simulink model "ServidorConNovint"  (Simulink 8.3)
settings: Solver=FixedStepDiscrete  StartTime=0.0  StopTime=inf  FixedStep=0.001  RelTol=1e-3
libraries: aerolibanimutils x1
settings Model: Creator=Usuario  LastModifiedBy=DdS
settings OptimizationCC: ExpressionDepthLimit=2147483647  SimCompilerOptimization=On
settings DebuggingCC: FcnCallInpInsideContextMsg=EnableAllAsWarning

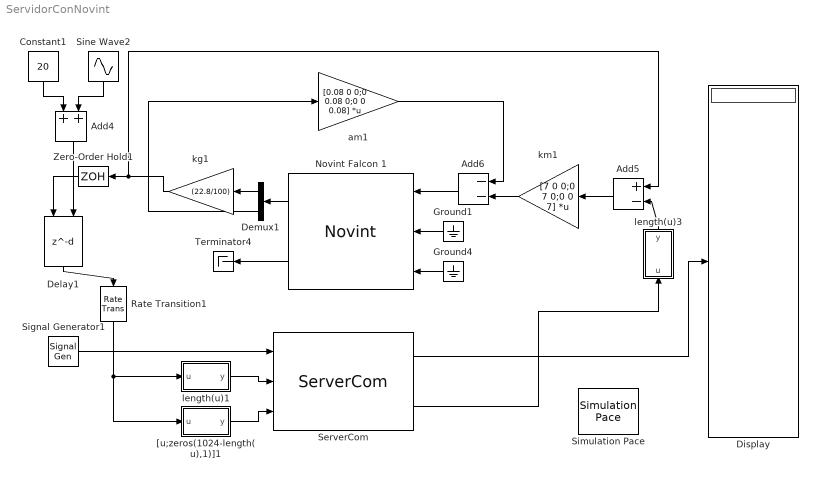
== system ServidorConNovint ==
  Add4 : Sum  SampleTime=0.05
  Add5 : Sum  Inputs=+-
  Add6 : Sum  Inputs=--
  Constant1 : Constant  Value=20  SampleTime=0.05
  Delay1 : Delay  DelayLengthSource=Input port  SampleTime=0.05
      settings: InputPortMap=u0,p1
  Demux1 : Demux  Outputs=[3 3]
  Display : Display
  Ground1 : Ground
  Ground4 : Ground
  Novint Falcon 1 : S-Function  FunctionName=Novint  Parameters=1  EnableBusSupport=off
      mask Display:
      | color('red')
      | port_label('input',1,'acciones')
      | port_label('input',2,'parametros')
      | port_label('input',3,'parametrosSend')
      | color('blue')
      | port_label('output',1,'estado')
      | port_label('output',2,'botones')
  Rate Transition1 : RateTransition  OutPortSampleTime=0
  ServerCom : S-Function  FunctionName=ServerCom  EnableBusSupport=off
      mask Display:
      | patch([0 4. 4 0],[0.02 0.02 0.98 0.98],0.9*[123 193 255]/255)
      | patch([0 4 4 0],[0.1 0.1 0.9 0.9],[123 193 255]/255)
      | patch([1.5 2.5 2.5 2.3 2.3 1.7 1.7 1.5],[0 0 1 1 1.2 1.2 1 1],[130 130 130]/255)
      | patch([1.3 2.7 2.7 1.3],[1.2 1.2 2.9 2.9],0.85*[130 130 130]/255)
      | patch([1.4 2.6 2.6 1.4],[1.3 1.3 2.8 2.8],[123 193 255]/255)
      | patch([1.5 2.5 2.5 1.5],[1.4 1.4 2.7 2.7],0.85*[130 130 130]/255)
      | patch([1.9 2.1 2.1 1.9],[1.8 1.8 2.1 2.1],[123 193 255]/255)
      | color('red')
      | port_label('input',1,'clock')
      | port_label('input',2,'sizeSend')
      | port_label('input',3,'dataSend')
      | port_label('output',1,'stateChannel')
      | port_label('output',2,'dataRecv')
  Signal Generator1 : SignalGenerator  WaveForm=square  Frequency=20
  Simulation Pace : aerolibanimutils/Simulation Pace  SimulationPace=1  SleepMode=MATLAB Thread  OutputPaceError=off  SampleTime=-1
      settings: AttributesFormatString=%<SimulationPace> sec/sec
  Sine Wave2 : Sin  Amplitude=0  Frequency=0.1*2*pi  SampleTime=0.05
  Terminator4 : Terminator
  Zero-Order Hold1 : ZeroOrderHold  SampleTime=0.05
  "[u;zeros(1024-length(u),1)]1" : MATLAB Function  TreatAsAtomicUnit=on
  am1 : Gain  Gain=[0.08 0 0;0 0.08 0;0 0 0.08]  Multiplication=Matrix(K*u)
  kg1 : Gain  Gain=(22.8/100)
  km1 : Gain  Gain=[7 0 0;0 7 0;0 0 7]  Multiplication=Matrix(K*u)
  length(u)1 : MATLAB Function  TreatAsAtomicUnit=on
  length(u)3 : MATLAB Function  TreatAsAtomicUnit=on
  wires:
  Signal Generator1/1 -> ServerCom/1
  length(u)1/1(y) -> ServerCom/2
  Novint Falcon 1/1 -> Demux1/1
  "[u;zeros(1024-length(u),1)]1"/1(y) -> ServerCom/3
  Novint Falcon 1/2 -> Terminator4/1
  ServerCom/1 -> Display/1
  ServerCom/2 -> length(u)3/1(u)
  Demux1/2 -> am1/1
  Add6/1 -> Novint Falcon 1/1
  Ground1/1 -> Novint Falcon 1/2
  Ground4/1 -> Novint Falcon 1/3
  Demux1/1 -> kg1/1
  kg1/1 -> Add5/1, Zero-Order Hold1/1
  Add5/1 -> km1/1
  km1/1 -> Add6/2
  Delay1/1 -> Rate Transition1/1
  Constant1/1 -> Add4/1
  Sine Wave2/1 -> Add4/2
  Add4/1 -> Delay1/2
  Zero-Order Hold1/1 -> Delay1/1
  Rate Transition1/1 -> length(u)1/1(u), "[u;zeros(1024-length(u),1)]1"/1(u)
  am1/1 -> Add6/1
  length(u)3/1(y) -> Add5/2

== matlab function [u;zeros(1024-length(u),1)]1 ==
  data: u input double; y output double
function y = fcn(u)
%#codegen

y = [u;zeros(1024-length(u),1)];

== matlab function length(u)1 ==
  data: u input double; y output double
function y = fcn(u)
%#codegen

y = uint32(length(u));

== matlab function length(u)3 ==
  data: u input double; y output double
function y = fcn(u)
%#codegen

y = u(1:3);
